simulink model "TI_OCEM_model"  (R2023a)
settings: Solver=ode23s  StartTime=0.0  StopTime=0.1  MaxStep=1e-4  RelTol=1e-3
libraries: spsGroundLib x2, spsSeriesRLCBranchLib x2, spsCurrentMeasurementLib x2, spsVoltageMeasurementLib x2, spsACCurrentSourceLib x1, spsSaturableTransformerLib x1, sps_lib x1
settings Model: Creator=KSSS  LastModifiedBy=KSSS
settings SolverCC: AlgebraicLoopSolver=TrustRegion
settings DataIOCC: ReturnWorkspaceOutputs=off
settings DebuggingCC: UnconnectedInputMsg=warning  UnconnectedOutputMsg=warning  UnconnectedLineMsg=warning  ArithmeticOperatorsInVariantConditions=warning
settings ModelReferenceCC: EnableRefExpFcnMdlSchedulingChecks=on
settings SFSimCC: SimUseLocalCustomCode=off  CustomCodeUndefinedFunction=UseInterfaceOnly
settings RTWCC: RTWUseLocalCustomCode=off
settings CodeAppCC: StateflowObjectComments=on
settings GRTTargetCC: CombineOutputUpdateFcns=off
settings SimscapeCC: SimscapeNormalizeSystem=off

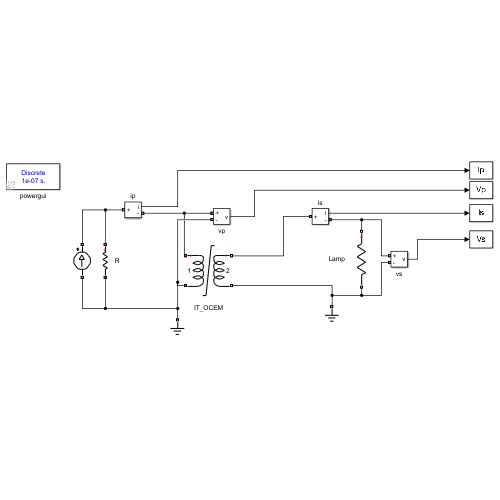
[thumbnail: Simulink's stored preview of the top-level diagram]
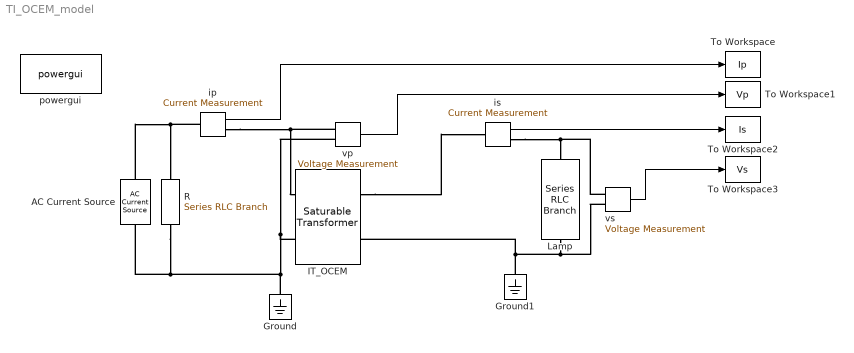
== system TI_OCEM_model ==
  AC Current Source : spsACCurrentSourceLib/AC Current Source  Amplitude=6.6*sqrt(2)  Phase=90  Frequency=50  SampleTime=0  Measurements=None
      settings: LibrarySourceBlock=sps_lib/Sources/AC Current Source
  Ground : spsGroundLib/Ground  LConnTagsString=a
  Ground1 : spsGroundLib/Ground  LConnTagsString=a
  IT_OCEM : spsSaturableTransformerLib/Saturable Transformer  ThreeWindings=off  Hysteresis=off  DataFile='hysteresis.mat'  Measurements=None  UNITS=SI  NominalPower=TI_OCEM.Pn_fn  Winding1=TI_OCEM.W1  Winding2=TI_OCEM.W2  Winding3=[3.15e+05 1.2118e+09 4.0926e+05]  Saturation=TI_OCEM.Sat  CoreLoss=TI_OCEM.Rm  BreakLoop=off  DiscreteSolver=Trapezoidal iterative  DataType=on  InitialFlux=0.0205600583592649  TransfoNumber=1
      settings: LibrarySourceBlock=sps_lib/Power Grid Elements/Saturable Transformer
  Lamp : spsSeriesRLCBranchLib/Series RLC Branch  LConnTagsString=__new0  RConnTagsString=__new0  BranchType=R  Resistance=6.887  Inductance=1e-3  SetiL0=off  InitialCurrent=0  Capacitance=1e-6  Setx0=off  InitialVoltage=0  Measurements=None
  R : spsSeriesRLCBranchLib/Series RLC Branch  LConnTagsString=__new0  RConnTagsString=__new0  BranchType=R  Resistance=1e8  Inductance=1e-3  SetiL0=off  InitialCurrent=0  Capacitance=1e-6  Setx0=off  InitialVoltage=0  Measurements=None
  To Workspace : ToWorkspace  VariableName=Ip  SaveFormat=Timeseries  SampleTime=-1
  To Workspace1 : ToWorkspace  VariableName=Vp  SaveFormat=Timeseries  SampleTime=-1
  To Workspace2 : ToWorkspace  VariableName=Is  SaveFormat=Timeseries  SampleTime=-1
  To Workspace3 : ToWorkspace  VariableName=Vs  SaveFormat=Timeseries  SampleTime=-1
  ip : spsCurrentMeasurementLib/Current Measurement  PhasorSimulation=off  OutputType=Complex  PSBequivalent=0
  is : spsCurrentMeasurementLib/Current Measurement  PhasorSimulation=off  OutputType=Complex  PSBequivalent=0
  powergui : sps_lib/powergui  Priority=1  SimulationMode=Discrete  SampleTime=10e-8  frequency=60  Iterations=50  frequencyindice=50  Pbase=100e6  ErrMax=1e-4  UnitsV=kV  UnitsW=MW  buscounter=0  FunctionMessages=off  echomessages=off  EnableUseOfTLC=off  CurrentSourceSwitches=on  DisableSnubberDevices=off  DisableRonSwitches=off  DisableVfSwitches=off  DisplayEquations=off  AutomaticDiscreteSolvers=off  SolverType=Tustin/Backward Euler (TBE)  Interpol=off  ExternalGateDelay=off  methode=off  Ts=100  x0status=blocks  SPID=on  SwTol=0  HookPort=off  NonlinearTolerance=1e-4  nMaxIteration=100  ContinueOnMaxIteration=off  RestoreLinks=warning  ResistiveCurrentMeasurement=off  Frange=[0:2:500]  Ylog=off  Xlog=on  ShowGrid=off  save=off  variable=ZData  structure=0  ZoomFFT=off  StartTime=0.0  cycles=1  DisplayStyle=1  fundamental=60  FreqAxis=off  MaxFrequency=1000  frequencyindicesteady=1  RmsSteady=1  display=off
  vp : spsVoltageMeasurementLib/Voltage Measurement  PhasorSimulation=off  OutputType=Complex  PSBequivalent=0
  vs : spsVoltageMeasurementLib/Voltage Measurement  PhasorSimulation=off  OutputType=Complex  PSBequivalent=0
  wires:
  ip/1 -> To Workspace/1
  vp/1 -> To Workspace1/1
  is/1 -> To Workspace2/1
  vs/1 -> To Workspace3/1
  connections:
  AC Current Source/RConn1 -- ip/LConn1 -- R/LConn1
  IT_OCEM/LConn2 -- vp/LConn2 -- Ground/LConn1 -- R/RConn1 -- AC Current Source/LConn1
  Lamp/RConn1 -- vs/LConn2 -- Ground1/LConn1 -- IT_OCEM/RConn2
  ip/RConn1 -- IT_OCEM/LConn1 -- vp/LConn1
  IT_OCEM/RConn1 -- is/LConn1
  is/RConn1 -- vs/LConn1 -- Lamp/LConn1
